simulink model "FunctionCallFeedbackLatch"  (R2017b)
settings: Solver=FixedStepDiscrete  StartTime=0.0  StopTime=100  FixedStep=0.200000  RelTol=1e-3
settings Model: Creator=hbourbou  LastModifiedBy=hbourbou
settings DataIOCC: ExternalInput=input_dataset  SaveState=on
settings DebuggingCC: AlgebraicLoopMsg=error  ArtificialAlgebraicLoopMsg=error  BlockPriorityViolationMsg=error  MinStepSizeMsg=error
settings GRTTargetCC: ExtMode=on

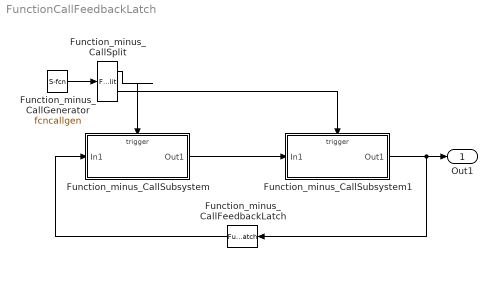
== system FunctionCallFeedbackLatch ==
  Function_minus_CallFeedbackLatch : FunctionCallFeedbackLatch
  Function_minus_CallGenerator : S-Function  AncestorBlock=|  FunctionName=fcncallgen  Parameters=sample_time,numberOfIterations  SFunctionDeploymentMode=off  EnableBusSupport=off  mask(Function-Call Generator){sample_time=1, numberOfIterations=1}
      | simulink/Ports &
      | Subsystems/Function-Call
      | Generator
      mask prompts: sample_time "Simulink:masks:SampleTime_MP"; numberOfIterations "Simulink:masks:NumberOfIterations_MP"
      mask help: Simulink:masks:FunctionCallGenerator_MD
      mask init:
      | if ~isempty(numberOfIterations) & length(numberOfIterations) == 1 & (numberOfIterations > 1),
      | str=sprintf('iterate I = 1:%d',numberOfIterations);
      | else, str = 'f()';
      | end;
      mask Help: This block executes a function-call subsystem at the rate specified by the sample time and a specified number of times.
      mask Display: disp(str)
  Function_minus_CallSplit : FunctionCallSplit  NumOutputPorts=2
  Function_minus_CallSubsystem : Subsystem  TreatAsAtomicUnit=on
  Function_minus_CallSubsystem1 : Subsystem  TreatAsAtomicUnit=on
  Out1 : Outport
  wires:
  Function_minus_CallSubsystem/1(Out1) -> Function_minus_CallSubsystem1/1(In1)
  Function_minus_CallGenerator/1 -> Function_minus_CallSplit/1
  Function_minus_CallSplit/1 -> Function_minus_CallSubsystem/Trigger
  Function_minus_CallSplit/2 -> Function_minus_CallSubsystem1/Trigger
  Function_minus_CallSubsystem1/1(Out1) -> Function_minus_CallFeedbackLatch/1, Out1/1
  Function_minus_CallFeedbackLatch/1 -> Function_minus_CallSubsystem/1(In1)

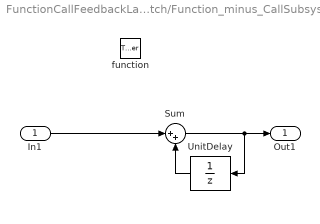
== system FunctionCallFeedbackLatch/Function_minus_CallSubsystem ==
  In1 : Inport
  function : TriggerPort  TriggerType=function-call  VariantControl=Variant
  Sum : Sum  Inputs=|++
  UnitDelay : UnitDelay  SampleTime=-1
  Out1 : Outport
  wires:
  In1/1 -> Sum/1
  Sum/1 -> UnitDelay/1, Out1/1
  UnitDelay/1 -> Sum/2

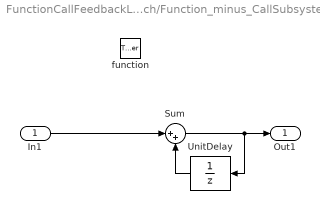
== system FunctionCallFeedbackLatch/Function_minus_CallSubsystem1 ==
  In1 : Inport
  function : TriggerPort  TriggerType=function-call  VariantControl=Variant
  Sum : Sum  Inputs=|++
  UnitDelay : UnitDelay  SampleTime=-1
  Out1 : Outport
  wires:
  In1/1 -> Sum/1
  Sum/1 -> UnitDelay/1, Out1/1
  UnitDelay/1 -> Sum/2
